simulink model "enable_1"  (Simulink 4.00)
settings: Solver=ode45  StartTime=0.0  StopTime=10.0  RelTol=1e-3
libraries: simulink3 x2
settings Model: LastModifiedBy=Administrator  BlockReductionOpt=off

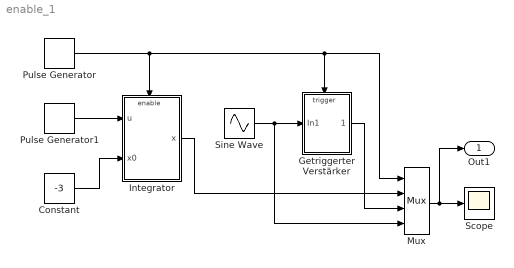
== system enable_1 ==
  Constant : Constant  Value=-3
  Getriggerter Verstärker : Subsystem  TreatAsAtomicUnit=on
      settings: RTWFcnNameOpts=Auto  RTWFileNameOpts=Auto
  Integrator : Subsystem  TreatAsAtomicUnit=on
      settings: RTWFcnNameOpts=Auto  RTWFileNameOpts=Auto
  Mux : Mux  Inputs=4
      settings: DisplayOption=none
  Pulse Generator : simulink3/Sources/Pulse Generator  period=1  duty=50  amplitude=1  start=0
  Pulse Generator1 : simulink3/Sources/Pulse Generator  period=1  duty=50  amplitude=1  start=0
  Scope : Scope
      settings: TimeRange=auto  YMin=-5  YMax=5  SaveToWorkspace=off  SaveName=ScopeData  LimitDataPoints=on  MaxDataPoints=5000
  Sine Wave : Sin  Amplitude=1  Frequency=1  Phase=0  SampleTime=0
  Out1 : Outport  Port=1
  wires:
  Pulse Generator1/1 -> Integrator/1(u)
  Constant/1 -> Integrator/2(x0)
  Pulse Generator/1 -> Integrator/Enable, Getriggerter Verstärker/Trigger, Mux/1
  Sine Wave/1 -> Getriggerter Verstärker/1(In1), Mux/4
  Integrator/1(x) -> Mux/2
  Getriggerter Verstärker/1(Out1) -> Mux/3
  Mux/1 -> Scope/1, Out1/1

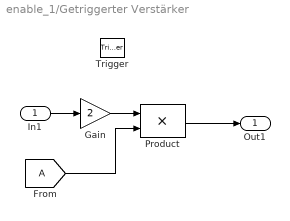
== system enable_1/Getriggerter Verstärker ==
  In1 : Inport  Port=1
  Trigger : TriggerPort  TriggerType=either  OutputDataType=auto
  Gain : Gain  Gain=2  Multiplication=Element-wise(K.*u)  SaturateOnIntegerOverflow=on
  Product : Product  Inputs=2  Multiplication=Element-wise(.*)  SaturateOnIntegerOverflow=on
  Out1 : Outport  Port=1
  wires:
  In1/1 -> Gain/1
  Gain/1 -> Product/1
  Product/1 -> Out1/1
  [A] -> Product/2

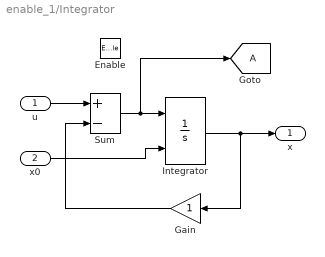
== system enable_1/Integrator ==
  u : Inport  Port=1
  x0 : Inport  Port=2
  Enable : EnablePort  StatesWhenEnabling=reset
  Gain : Gain  Orientation=left  Gain=1  Multiplication=Element-wise(K.*u)  SaturateOnIntegerOverflow=on
  Integrator : Integrator  ExternalReset=none  InitialConditionSource=external  InitialCondition=0  LimitOutput=off  UpperSaturationLimit=inf  LowerSaturationLimit=-inf  ShowSaturationPort=off  ShowStatePort=off  AbsoluteTolerance=auto
  Sum : Sum  Inputs=+-  SaturateOnIntegerOverflow=on
  x : Outport  Port=1
  tag scope: A=global
  wires:
  u/1 -> Sum/1
  Sum/1 -> Integrator/1, [A]
  x0/1 -> Integrator/2
  Gain/1 -> Sum/2
  Integrator/1 -> Gain/1, x/1
